simulink model "error_dynamics_simulink"  (R2020b)
settings: Solver=FixedStepAuto  StartTime=0.0  StopTime=10.0  FixedStep=1e-3  RelTol=1e-3
StartFcn:
  | m = 1;
  | k = 25;
  | b = 20;
settings Model: Creator=a302  LastModifiedBy=a302
settings RTWCC: Description=Create Visual C/C++ Solution File for Simulink Coder  TemplateMakefile=RTW.MSVCBuild

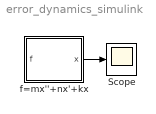
== system error_dynamics_simulink ==
  Scope : Scope
  f=mx''+nx'+kx : Subsystem  mask{k=1, b=1, m=1, x0=1, dx0=0}
  wires:
  f=mx''+nx'+kx/1(x) -> Scope/1

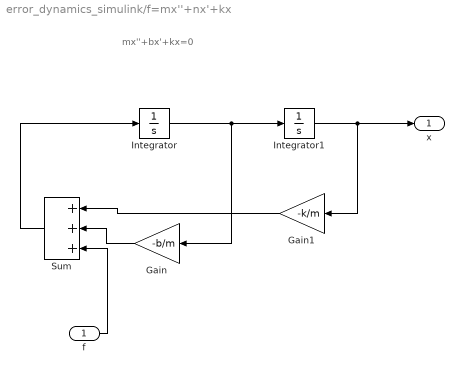
== system error_dynamics_simulink/f=mx''+nx'+kx ==
  note: mx''+bx'+kx=0
  f : Inport
  Gain : Gain  Gain=-b/m
  Gain1 : Gain  Gain=-k/m
  Integrator : Integrator  InitialCondition=dx0
  Integrator1 : Integrator  InitialCondition=x0
  Sum : Sum  Inputs=+++
  x : Outport
  wires:
  Integrator1/1 -> x/1, Gain1/1
  Integrator/1 -> Gain/1, Integrator1/1
  Gain1/1 -> Sum/1
  Sum/1 -> Integrator/1
  Gain/1 -> Sum/2
  f/1 -> Sum/3
